simulink model "untitled"  (R2017b)
settings: Solver=VariableStepAuto  StartTime=0.0  StopTime=10.0  RelTol=1e-3
settings Model: Creator=DELL-PC  LastModifiedBy=DELL-PC

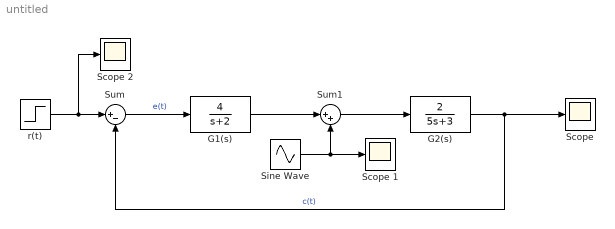
== system untitled ==
  G1(s) : TransferFcn  Numerator=[4]  Denominator=[1 2]
  G2(s) : TransferFcn  Numerator=[2]  Denominator=[5 3]
  "Scope " : Scope
  Scope 1 : Scope
  Scope 2 : Scope
  Sine Wave : Sin  TimeSource=Use external signal  Amplitude=0.1  Frequency=1000  SampleTime=0
  Sum : Sum  Inputs=|+-
  Sum1 : Sum  Inputs=|++
  "r(t) " : Step  Time=0  After=2  SampleTime=0
  wires:
  "r(t) "/1 -> Scope 2/1, Sum/1
  Sum/1 -> G1(s)/1  "e(t)"
  G2(s)/1 -> Sum/2, "Scope "/1  "c(t)"
  G1(s)/1 -> Sum1/1
  Sum1/1 -> G2(s)/1
  Sine Wave/1 -> Scope 1/1, Sum1/2
